simulink model "draft3"  (R2023a)
settings: Solver=VariableStepAuto  StartTime=0.0  StopTime=inf  FixedStep=0.0001  MaxStep=0.2  RelTol=1e-3  AbsTol=1e-3  EnableMultiTasking=on
model workspace (MAT data in the model file):
  c = 0.1
  k : Simulink.Parameter (value not decoded)
libraries: sm_lib x40, nesl_utility x35, simulink_extras x2, fl_lib x1
(part 2 of 3)

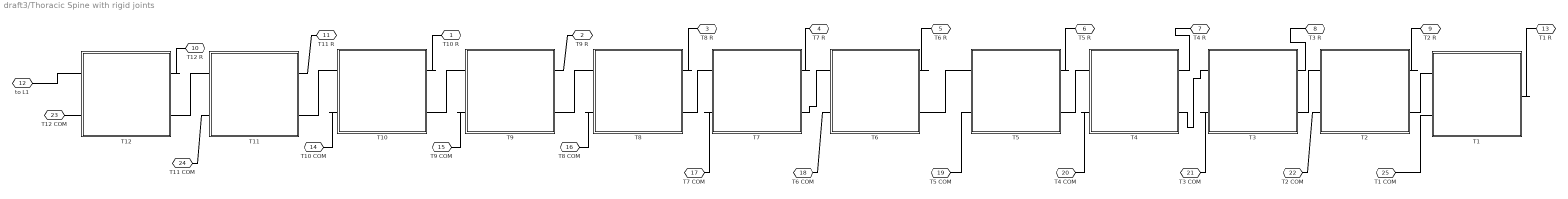
== system draft3/Thoracic Spine with rigid joints ==
  T1 : Subsystem
  T10 : Subsystem
  T11 : Subsystem
  T12 : Subsystem
  T2 : Subsystem
  T3 : Subsystem
  T4 : Subsystem
  T5 : Subsystem
  T6 : Subsystem
  T7 : Subsystem
  T8 : Subsystem
  T9 : Subsystem
  T10 R : PMIOPort  Side=Right
  T9 R : PMIOPort  Port=2  Side=Right
  T8 R : PMIOPort  Port=3  Side=Right
  T7 R : PMIOPort  Port=4  Side=Right
  T6 R : PMIOPort  Port=5  Side=Right
  T5 R : PMIOPort  Port=6  Side=Right
  T4 R : PMIOPort  Port=7  Side=Right
  T3 R : PMIOPort  Port=8  Side=Right
  T2 R : PMIOPort  Port=9  Side=Right
  T12 R : PMIOPort  Port=10  Side=Right
  T11 R : PMIOPort  Port=11  Side=Right
  to L1 : PMIOPort  Port=12  Side=Left
  T1 R : PMIOPort  Port=13  Side=Right
  T10 COM : PMIOPort  Port=14  Side=Left
  T9 COM : PMIOPort  Port=15  Side=Left
  T8 COM : PMIOPort  Port=16  Side=Left
  T7 COM : PMIOPort  Port=17  Side=Left
  T6 COM : PMIOPort  Port=18  Side=Left
  T5 COM : PMIOPort  Port=19  Side=Left
  T4 COM : PMIOPort  Port=20  Side=Left
  T3 COM : PMIOPort  Port=21  Side=Left
  T2 COM : PMIOPort  Port=22  Side=Left
  T12 COM : PMIOPort  Port=23  Side=Left
  T11 COM : PMIOPort  Port=24  Side=Left
  T1 COM : PMIOPort  Port=25  Side=Left
  connections:
  T4/LConn2 -- T4 COM/RConn1
  T7/LConn1 -- T8/RConn2
  T7/LConn2 -- T7 COM/RConn1
  T11/LConn2 -- T11 COM/RConn1
  T1/LConn1 -- T2/RConn2
  T8/LConn1 -- T9/RConn2
  T9/RConn1 -- T9 R/RConn1
  T11/RConn1 -- T11 R/RConn1
  T10/LConn1 -- T11/RConn2
  T5/LConn1 -- T6/RConn2
  T9/LConn1 -- T10/RConn2
  T12/RConn1 -- T12 R/RConn1
  T11/LConn1 -- T12/RConn2
  T1/LConn2 -- T1 COM/RConn1
  T8/LConn2 -- T8 COM/RConn1
  T5/LConn2 -- T5 COM/RConn1
  T6/LConn1 -- T7/RConn2
  T2/LConn2 -- T2 COM/RConn1
  T4/RConn2 -- T3/LConn1
  T10/RConn1 -- T10 R/RConn1
  T2/LConn1 -- T3/RConn2
  T1/RConn1 -- T1 R/RConn1
  T4/LConn1 -- T5/RConn2
  T3/LConn2 -- T3 COM/RConn1
  T12/LConn1 -- to L1/RConn1
  T3/RConn1 -- T3 R/RConn1
  T5/RConn1 -- T5 R/RConn1
  T7/RConn1 -- T7 R/RConn1
  T12/LConn2 -- T12 COM/RConn1
  T2/RConn1 -- T2 R/RConn1
  T6/LConn2 -- T6 COM/RConn1
  T6/RConn1 -- T6 R/RConn1
  T10/LConn2 -- T10 COM/RConn1
  T9/LConn2 -- T9 COM/RConn1
  T4/RConn1 -- T4 R/RConn1
  T8/RConn1 -- T8 R/RConn1

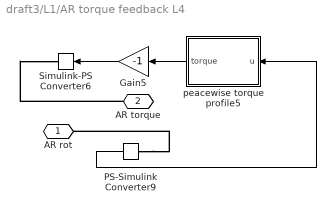
== system draft3/L1/AR torque feedback L4 ==
  Gain5 : Gain  Gain=-1
  PS-Simulink Converter9 : nesl_utility/PS-Simulink Converter  PhysicalDomain=network_engine_domain  SubClassName=ps_output  LeftPortType=input  RightPortType=output  PseudoPeriodic=off  Frequencies=[]  VectorFormat=1-D array  Unit=inherit  AffineConversion=off
  Simulink-PS Converter6 : nesl_utility/Simulink-PS Converter  PhysicalDomain=network_engine_domain  SubClassName=ps_input  LeftPortType=input  RightPortType=output  PseudoPeriodic=off  Frequencies=[]  NoiseDistribution=none  NoiseParameters=[]  Unit=1  AffineConversion=off  FilteringAndDerivatives=provide  SimscapeFilterOrder=1  InputFilterTimeConstant=0.001  UdotUserProvided=0
  peacewise torque profile5 : MATLAB Function  TreatAsAtomicUnit=on
  AR rot : PMIOPort  Side=Left
  AR torque : PMIOPort  Port=2  Side=Right
  wires:
  PS-Simulink Converter9/1 -> peacewise torque profile5/1(u)
  peacewise torque profile5/1(torque) -> Gain5/1
  Gain5/1 -> Simulink-PS Converter6/1
  connections:
  PS-Simulink Converter9/LConn1 -- AR rot/RConn1
  AR torque/RConn1 -- Simulink-PS Converter6/RConn1

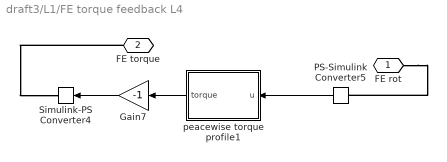
== system draft3/L1/FE torque feedback L4 ==
  Gain7 : Gain  Gain=-1
  PS-Simulink Converter5 : nesl_utility/PS-Simulink Converter  PhysicalDomain=network_engine_domain  SubClassName=ps_output  LeftPortType=input  RightPortType=output  PseudoPeriodic=off  Frequencies=[]  VectorFormat=1-D array  Unit=inherit  AffineConversion=off
  Simulink-PS Converter4 : nesl_utility/Simulink-PS Converter  PhysicalDomain=network_engine_domain  SubClassName=ps_input  LeftPortType=input  RightPortType=output  PseudoPeriodic=off  Frequencies=[]  NoiseDistribution=none  NoiseParameters=[]  Unit=1  AffineConversion=off  FilteringAndDerivatives=provide  SimscapeFilterOrder=1  InputFilterTimeConstant=0.001  UdotUserProvided=0
  peacewise torque profile1 : MATLAB Function  TreatAsAtomicUnit=on
  FE rot : PMIOPort  Side=Left
  FE torque : PMIOPort  Port=2  Side=Right
  wires:
  PS-Simulink Converter5/1 -> peacewise torque profile1/1(u)
  peacewise torque profile1/1(torque) -> Gain7/1
  Gain7/1 -> Simulink-PS Converter4/1
  connections:
  FE rot/RConn1 -- PS-Simulink Converter5/LConn1
  FE torque/RConn1 -- Simulink-PS Converter4/RConn1

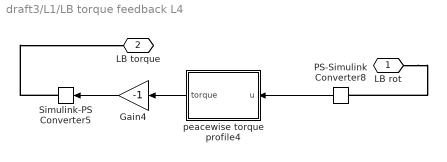
== system draft3/L1/LB torque feedback L4 ==
  Gain4 : Gain  Gain=-1
  PS-Simulink Converter8 : nesl_utility/PS-Simulink Converter  PhysicalDomain=network_engine_domain  SubClassName=ps_output  LeftPortType=input  RightPortType=output  PseudoPeriodic=off  Frequencies=[]  VectorFormat=1-D array  Unit=inherit  AffineConversion=off
  Simulink-PS Converter5 : nesl_utility/Simulink-PS Converter  PhysicalDomain=network_engine_domain  SubClassName=ps_input  LeftPortType=input  RightPortType=output  PseudoPeriodic=off  Frequencies=[]  NoiseDistribution=none  NoiseParameters=[]  Unit=1  AffineConversion=off  FilteringAndDerivatives=provide  SimscapeFilterOrder=1  InputFilterTimeConstant=0.001  UdotUserProvided=0
  peacewise torque profile4 : MATLAB Function  TreatAsAtomicUnit=on
  LB rot : PMIOPort  Side=Left
  LB torque : PMIOPort  Port=2  Side=Right
  wires:
  Gain4/1 -> Simulink-PS Converter5/1
  PS-Simulink Converter8/1 -> peacewise torque profile4/1(u)
  peacewise torque profile4/1(torque) -> Gain4/1
  connections:
  Simulink-PS Converter5/RConn1 -- LB torque/RConn1
  LB rot/RConn1 -- PS-Simulink Converter8/LConn1

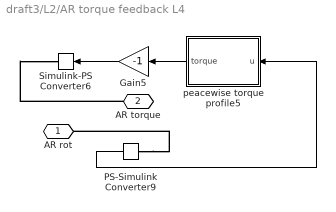
== system draft3/L2/AR torque feedback L4 ==
  Gain5 : Gain  Gain=-1
  PS-Simulink Converter9 : nesl_utility/PS-Simulink Converter  PhysicalDomain=network_engine_domain  SubClassName=ps_output  LeftPortType=input  RightPortType=output  PseudoPeriodic=off  Frequencies=[]  VectorFormat=1-D array  Unit=inherit  AffineConversion=off
  Simulink-PS Converter6 : nesl_utility/Simulink-PS Converter  PhysicalDomain=network_engine_domain  SubClassName=ps_input  LeftPortType=input  RightPortType=output  PseudoPeriodic=off  Frequencies=[]  NoiseDistribution=none  NoiseParameters=[]  Unit=1  AffineConversion=off  FilteringAndDerivatives=provide  SimscapeFilterOrder=1  InputFilterTimeConstant=0.001  UdotUserProvided=0
  peacewise torque profile5 : MATLAB Function  TreatAsAtomicUnit=on
  AR rot : PMIOPort  Side=Left
  AR torque : PMIOPort  Port=2  Side=Right
  wires:
  Gain5/1 -> Simulink-PS Converter6/1
  peacewise torque profile5/1(torque) -> Gain5/1
  PS-Simulink Converter9/1 -> peacewise torque profile5/1(u)
  connections:
  AR torque/RConn1 -- Simulink-PS Converter6/RConn1
  PS-Simulink Converter9/LConn1 -- AR rot/RConn1

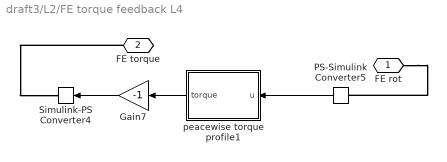
== system draft3/L2/FE torque feedback L4 ==
  Gain7 : Gain  Gain=-1
  PS-Simulink Converter5 : nesl_utility/PS-Simulink Converter  PhysicalDomain=network_engine_domain  SubClassName=ps_output  LeftPortType=input  RightPortType=output  PseudoPeriodic=off  Frequencies=[]  VectorFormat=1-D array  Unit=inherit  AffineConversion=off
  Simulink-PS Converter4 : nesl_utility/Simulink-PS Converter  PhysicalDomain=network_engine_domain  SubClassName=ps_input  LeftPortType=input  RightPortType=output  PseudoPeriodic=off  Frequencies=[]  NoiseDistribution=none  NoiseParameters=[]  Unit=1  AffineConversion=off  FilteringAndDerivatives=provide  SimscapeFilterOrder=1  InputFilterTimeConstant=0.001  UdotUserProvided=0
  peacewise torque profile1 : MATLAB Function  TreatAsAtomicUnit=on
  FE rot : PMIOPort  Side=Left
  FE torque : PMIOPort  Port=2  Side=Right
  wires:
  Gain7/1 -> Simulink-PS Converter4/1
  peacewise torque profile1/1(torque) -> Gain7/1
  PS-Simulink Converter5/1 -> peacewise torque profile1/1(u)
  connections:
  FE torque/RConn1 -- Simulink-PS Converter4/RConn1
  FE rot/RConn1 -- PS-Simulink Converter5/LConn1

== system draft3/L2/LB torque feedback L4 ==
  Gain4 : Gain  Gain=-1
  PS-Simulink Converter8 : nesl_utility/PS-Simulink Converter  PhysicalDomain=network_engine_domain  SubClassName=ps_output  LeftPortType=input  RightPortType=output  PseudoPeriodic=off  Frequencies=[]  VectorFormat=1-D array  Unit=inherit  AffineConversion=off
  Simulink-PS Converter5 : nesl_utility/Simulink-PS Converter  PhysicalDomain=network_engine_domain  SubClassName=ps_input  LeftPortType=input  RightPortType=output  PseudoPeriodic=off  Frequencies=[]  NoiseDistribution=none  NoiseParameters=[]  Unit=1  AffineConversion=off  FilteringAndDerivatives=provide  SimscapeFilterOrder=1  InputFilterTimeConstant=0.001  UdotUserProvided=0
  peacewise torque profile4 : MATLAB Function  TreatAsAtomicUnit=on
  LB rot : PMIOPort  Side=Left
  LB torque : PMIOPort  Port=2  Side=Right
  wires:
  peacewise torque profile4/1(torque) -> Gain4/1
  PS-Simulink Converter8/1 -> peacewise torque profile4/1(u)
  Gain4/1 -> Simulink-PS Converter5/1
  connections:
  LB rot/RConn1 -- PS-Simulink Converter8/LConn1
  Simulink-PS Converter5/RConn1 -- LB torque/RConn1

== system draft3/L3/AR torque feedback L4 ==
  Gain5 : Gain  Gain=-1
  PS-Simulink Converter9 : nesl_utility/PS-Simulink Converter  PhysicalDomain=network_engine_domain  SubClassName=ps_output  LeftPortType=input  RightPortType=output  PseudoPeriodic=off  Frequencies=[]  VectorFormat=1-D array  Unit=inherit  AffineConversion=off
  Simulink-PS Converter6 : nesl_utility/Simulink-PS Converter  PhysicalDomain=network_engine_domain  SubClassName=ps_input  LeftPortType=input  RightPortType=output  PseudoPeriodic=off  Frequencies=[]  NoiseDistribution=none  NoiseParameters=[]  Unit=1  AffineConversion=off  FilteringAndDerivatives=provide  SimscapeFilterOrder=1  InputFilterTimeConstant=0.001  UdotUserProvided=0
  peacewise torque profile5 : MATLAB Function  TreatAsAtomicUnit=on
  AR rot : PMIOPort  Side=Left
  AR torque : PMIOPort  Port=2  Side=Right
  wires:
  PS-Simulink Converter9/1 -> peacewise torque profile5/1(u)
  peacewise torque profile5/1(torque) -> Gain5/1
  Gain5/1 -> Simulink-PS Converter6/1
  connections:
  PS-Simulink Converter9/LConn1 -- AR rot/RConn1
  AR torque/RConn1 -- Simulink-PS Converter6/RConn1

== system draft3/L3/FE torque feedback L4 ==
  Gain7 : Gain  Gain=-1
  PS-Simulink Converter5 : nesl_utility/PS-Simulink Converter  PhysicalDomain=network_engine_domain  SubClassName=ps_output  LeftPortType=input  RightPortType=output  PseudoPeriodic=off  Frequencies=[]  VectorFormat=1-D array  Unit=inherit  AffineConversion=off
  Simulink-PS Converter4 : nesl_utility/Simulink-PS Converter  PhysicalDomain=network_engine_domain  SubClassName=ps_input  LeftPortType=input  RightPortType=output  PseudoPeriodic=off  Frequencies=[]  NoiseDistribution=none  NoiseParameters=[]  Unit=1  AffineConversion=off  FilteringAndDerivatives=provide  SimscapeFilterOrder=1  InputFilterTimeConstant=0.001  UdotUserProvided=0
  peacewise torque profile1 : MATLAB Function  TreatAsAtomicUnit=on
  FE rot : PMIOPort  Side=Left
  FE torque : PMIOPort  Port=2  Side=Right
  wires:
  PS-Simulink Converter5/1 -> peacewise torque profile1/1(u)
  peacewise torque profile1/1(torque) -> Gain7/1
  Gain7/1 -> Simulink-PS Converter4/1
  connections:
  FE rot/RConn1 -- PS-Simulink Converter5/LConn1
  FE torque/RConn1 -- Simulink-PS Converter4/RConn1

== system draft3/L3/LB torque feedback L4 ==
  Gain4 : Gain  Gain=-1
  PS-Simulink Converter8 : nesl_utility/PS-Simulink Converter  PhysicalDomain=network_engine_domain  SubClassName=ps_output  LeftPortType=input  RightPortType=output  PseudoPeriodic=off  Frequencies=[]  VectorFormat=1-D array  Unit=inherit  AffineConversion=off
  Simulink-PS Converter5 : nesl_utility/Simulink-PS Converter  PhysicalDomain=network_engine_domain  SubClassName=ps_input  LeftPortType=input  RightPortType=output  PseudoPeriodic=off  Frequencies=[]  NoiseDistribution=none  NoiseParameters=[]  Unit=1  AffineConversion=off  FilteringAndDerivatives=provide  SimscapeFilterOrder=1  InputFilterTimeConstant=0.001  UdotUserProvided=0
  peacewise torque profile4 : MATLAB Function  TreatAsAtomicUnit=on
  LB rot : PMIOPort  Side=Left
  LB torque : PMIOPort  Port=2  Side=Right
  wires:
  Gain4/1 -> Simulink-PS Converter5/1
  PS-Simulink Converter8/1 -> peacewise torque profile4/1(u)
  peacewise torque profile4/1(torque) -> Gain4/1
  connections:
  Simulink-PS Converter5/RConn1 -- LB torque/RConn1
  LB rot/RConn1 -- PS-Simulink Converter8/LConn1

== system draft3/L4/AR torque feedback L4 ==
  Gain5 : Gain  Gain=-1
  PS-Simulink Converter9 : nesl_utility/PS-Simulink Converter  PhysicalDomain=network_engine_domain  SubClassName=ps_output  LeftPortType=input  RightPortType=output  PseudoPeriodic=off  Frequencies=[]  VectorFormat=1-D array  Unit=inherit  AffineConversion=off
  Simulink-PS Converter6 : nesl_utility/Simulink-PS Converter  PhysicalDomain=network_engine_domain  SubClassName=ps_input  LeftPortType=input  RightPortType=output  PseudoPeriodic=off  Frequencies=[]  NoiseDistribution=none  NoiseParameters=[]  Unit=1  AffineConversion=off  FilteringAndDerivatives=provide  SimscapeFilterOrder=1  InputFilterTimeConstant=0.001  UdotUserProvided=0
  peacewise torque profile5 : MATLAB Function  TreatAsAtomicUnit=on
  AR rot : PMIOPort  Side=Left
  AR torque : PMIOPort  Port=2  Side=Right
  wires:
  Gain5/1 -> Simulink-PS Converter6/1
  peacewise torque profile5/1(torque) -> Gain5/1
  PS-Simulink Converter9/1 -> peacewise torque profile5/1(u)
  connections:
  AR torque/RConn1 -- Simulink-PS Converter6/RConn1
  PS-Simulink Converter9/LConn1 -- AR rot/RConn1

== system draft3/L4/FE torque feedback L4 ==
  Gain7 : Gain  Gain=-1
  PS-Simulink Converter5 : nesl_utility/PS-Simulink Converter  PhysicalDomain=network_engine_domain  SubClassName=ps_output  LeftPortType=input  RightPortType=output  PseudoPeriodic=off  Frequencies=[]  VectorFormat=1-D array  Unit=inherit  AffineConversion=off
  Simulink-PS Converter4 : nesl_utility/Simulink-PS Converter  PhysicalDomain=network_engine_domain  SubClassName=ps_input  LeftPortType=input  RightPortType=output  PseudoPeriodic=off  Frequencies=[]  NoiseDistribution=none  NoiseParameters=[]  Unit=1  AffineConversion=off  FilteringAndDerivatives=provide  SimscapeFilterOrder=1  InputFilterTimeConstant=0.001  UdotUserProvided=0
  peacewise torque profile1 : MATLAB Function  TreatAsAtomicUnit=on
  FE rot : PMIOPort  Side=Left
  FE torque : PMIOPort  Port=2  Side=Right
  wires:
  Gain7/1 -> Simulink-PS Converter4/1
  peacewise torque profile1/1(torque) -> Gain7/1
  PS-Simulink Converter5/1 -> peacewise torque profile1/1(u)
  connections:
  FE torque/RConn1 -- Simulink-PS Converter4/RConn1
  FE rot/RConn1 -- PS-Simulink Converter5/LConn1

== system draft3/L4/LB torque feedback L4 ==
  Gain4 : Gain  Gain=-1
  PS-Simulink Converter8 : nesl_utility/PS-Simulink Converter  PhysicalDomain=network_engine_domain  SubClassName=ps_output  LeftPortType=input  RightPortType=output  PseudoPeriodic=off  Frequencies=[]  VectorFormat=1-D array  Unit=inherit  AffineConversion=off
  Simulink-PS Converter5 : nesl_utility/Simulink-PS Converter  PhysicalDomain=network_engine_domain  SubClassName=ps_input  LeftPortType=input  RightPortType=output  PseudoPeriodic=off  Frequencies=[]  NoiseDistribution=none  NoiseParameters=[]  Unit=1  AffineConversion=off  FilteringAndDerivatives=provide  SimscapeFilterOrder=1  InputFilterTimeConstant=0.001  UdotUserProvided=0
  peacewise torque profile4 : MATLAB Function  TreatAsAtomicUnit=on
  LB rot : PMIOPort  Side=Left
  LB torque : PMIOPort  Port=2  Side=Right
  wires:
  peacewise torque profile4/1(torque) -> Gain4/1
  PS-Simulink Converter8/1 -> peacewise torque profile4/1(u)
  Gain4/1 -> Simulink-PS Converter5/1
  connections:
  LB rot/RConn1 -- PS-Simulink Converter8/LConn1
  Simulink-PS Converter5/RConn1 -- LB torque/RConn1

== system draft3/L5/AR torque feedback L5 ==
  Gain2 : Gain  Gain=-1
  PS-Simulink Converter3 : nesl_utility/PS-Simulink Converter  PhysicalDomain=network_engine_domain  SubClassName=ps_output  LeftPortType=input  RightPortType=output  PseudoPeriodic=off  Frequencies=[]  VectorFormat=1-D array  Unit=inherit  AffineConversion=off
  Simulink-PS Converter2 : nesl_utility/Simulink-PS Converter  PhysicalDomain=network_engine_domain  SubClassName=ps_input  LeftPortType=input  RightPortType=output  PseudoPeriodic=off  Frequencies=[]  NoiseDistribution=none  NoiseParameters=[]  Unit=1  AffineConversion=off  FilteringAndDerivatives=provide  SimscapeFilterOrder=1  InputFilterTimeConstant=0.001  UdotUserProvided=0
  peacewise torque profile3 : MATLAB Function  TreatAsAtomicUnit=on
  AR rot : PMIOPort  Side=Left
  AR torque : PMIOPort  Port=2  Side=Right
  wires:
  peacewise torque profile3/1(torque) -> Gain2/1
  Gain2/1 -> Simulink-PS Converter2/1
  PS-Simulink Converter3/1 -> peacewise torque profile3/1(u)
  connections:
  AR torque/RConn1 -- Simulink-PS Converter2/RConn1
  PS-Simulink Converter3/LConn1 -- AR rot/RConn1

== system draft3/L5/FE torque feedback L5 ==
  Gain6 : Gain  Gain=-1
  PS-Simulink Converter1 : nesl_utility/PS-Simulink Converter  PhysicalDomain=network_engine_domain  SubClassName=ps_output  LeftPortType=input  RightPortType=output  PseudoPeriodic=off  Frequencies=[]  VectorFormat=1-D array  Unit=inherit  AffineConversion=off
  Simulink-PS Converter3 : nesl_utility/Simulink-PS Converter  PhysicalDomain=network_engine_domain  SubClassName=ps_input  LeftPortType=input  RightPortType=output  PseudoPeriodic=off  Frequencies=[]  NoiseDistribution=none  NoiseParameters=[]  Unit=1  AffineConversion=off  FilteringAndDerivatives=provide  SimscapeFilterOrder=1  InputFilterTimeConstant=0.001  UdotUserProvided=0
  peacewise torque profile (+- 15 deg) : MATLAB Function  TreatAsAtomicUnit=on
  FE torque : PMIOPort  Side=Right
  FE rot : PMIOPort  Port=2  Side=Left
  wires:
  Gain6/1 -> Simulink-PS Converter3/1
  PS-Simulink Converter1/1 -> peacewise torque profile (+- 15 deg)/1(u)
  peacewise torque profile (+- 15 deg)/1(torque) -> Gain6/1
  connections:
  PS-Simulink Converter1/LConn1 -- FE rot/RConn1
  Simulink-PS Converter3/RConn1 -- FE torque/RConn1

== system draft3/L5/LB torque feedback L5 ==
  Gain1 : Gain  Gain=-1
  PS-Simulink Converter2 : nesl_utility/PS-Simulink Converter  PhysicalDomain=network_engine_domain  SubClassName=ps_output  LeftPortType=input  RightPortType=output  PseudoPeriodic=off  Frequencies=[]  VectorFormat=1-D array  Unit=inherit  AffineConversion=off
  Simulink-PS Converter1 : nesl_utility/Simulink-PS Converter  PhysicalDomain=network_engine_domain  SubClassName=ps_input  LeftPortType=input  RightPortType=output  PseudoPeriodic=off  Frequencies=[]  NoiseDistribution=none  NoiseParameters=[]  Unit=1  AffineConversion=off  FilteringAndDerivatives=provide  SimscapeFilterOrder=1  InputFilterTimeConstant=0.001  UdotUserProvided=0
  peacewise torque profile2 : MATLAB Function  TreatAsAtomicUnit=on
  LB rot : PMIOPort  Side=Left
  LB torque : PMIOPort  Port=2  Side=Right
  wires:
  Gain1/1 -> Simulink-PS Converter1/1
  PS-Simulink Converter2/1 -> peacewise torque profile2/1(u)
  peacewise torque profile2/1(torque) -> Gain1/1
  connections:
  LB rot/RConn1 -- PS-Simulink Converter2/LConn1
  Simulink-PS Converter1/RConn1 -- LB torque/RConn1

== system draft3/Thoracic Spine with rigid joints/T1 ==
  T1 : sm_lib/Body Elements/File Solid  ExtGeomFileName=C:\Users\siril\OneDrive\Desktop\TIM-Control\Matlab\Simscape models\CAD - with COM\T1_.step  UnitType=FromFile  ExtGeomFileUnits=m  StepReaderType=HEX  ExportConvexHullGeometry=off  InertiaType=CalculateFromGeometry  Mass=1  MassUnits=kg  CenterOfMass=[0 0 0]  CenterOfMassUnits=m  MomentsOfInertia=[1 1 1]  MomentsOfInertiaUnits=kg*m^2  ProductsOfInertia=[0 0 0]  ProductsOfInertiaUnits=kg*m^2  BasedOnType=Density  Density=0.99  DensityUnits=g/cm^3  DoExposeReferenceFrame=on  SerializedFrames=<Frames><Frame><Id>Frame1</Id><Value><Name>COM</Name><Origin><Source>CenterOfMassFrame</Source><FeatureName></FeatureName></Origin><PrimaryAxis><DefinedDirection>+Z</DefinedDirection><Source>ReferenceFrame</Source><SourceDirection>+Z</SourceDirection><FeatureName></FeatureName></PrimaryAxis><SecondaryAxis><DefinedDirection>+X</DefinedDirection><Source>ReferenceFrame</Source><SourceDirection>+X</SourceDirection><FeatureName></FeatureName></SecondaryAxis></Value></Frame><Frame><Id>Frame2</Id><Value><Name>to T2</Name><Origin><Source>GeometricFeature</Source><FeatureName>planar surface 5</FeatureName></Origin><PrimaryAxis><DefinedDirection>+X</DefinedDirection><Source>GeometricFeature</Source><SourceDirection>+Z</SourceDirection><FeatureName>planar surface 5</FeatureName></PrimaryAxis><SecondaryAxis><DefinedDirection>+Y</DefinedDirection><Source>ReferenceFrame</Source><SourceDirection>+X</SourceDirection><FeatureName></FeatureName></SecondaryAxis></Value></Frame></Frames>  GraphicType=FromGeometry  MarkerShape=Sphere  MarkerSize=10  GraphicVisPropType=SimpleVisualProperties  GraphicDiffuseColor=[0.5 0.5 0.5]  GraphicSpecularColor=[0.5 0.5 0.5 1.0]  GraphicAmbientColor=[0.15 0.15 0.15 1.0]  GraphicEmissiveColor=[0.0 0.0 0.0 1.0]  GraphicShininess=75  GraphicOpacity=1.0
  Weld Joint : sm_lib/Joints/Weld Joint  JointMode=Normal  SenseConstraintForce=off  SenseConstraintForceX=off  SenseConstraintForceY=off  SenseConstraintForceZ=off  SenseConstraintTorque=off  SenseConstraintTorqueX=off  SenseConstraintTorqueY=off  SenseConstraintTorqueZ=off  SenseTotalForce=off  SenseTotalForceX=off  SenseTotalForceY=off  SenseTotalForceZ=off  SenseTotalTorque=off  SenseTotalTorqueX=off  SenseTotalTorqueY=off  SenseTotalTorqueZ=off  CompositeWrenchDir=FollowerOnBase  CompositeWrenchFrame=BaseFrame
  to T2 : PMIOPort  Side=Left
  T1 COM : PMIOPort  Port=2  Side=Left
  T1 R : PMIOPort  Port=3  Side=Right
  connections:
  Weld Joint/LConn1 -- to T2/RConn1
  T1 COM/RConn1 -- T1/LConn1
  Weld Joint/RConn1 -- T1/LConn2
  T1/RConn1 -- T1 R/RConn1

== system draft3/Thoracic Spine with rigid joints/T10 ==
  T10 : sm_lib/Body Elements/File Solid  ExtGeomFileName=C:\Users\siril\OneDrive\Desktop\TIM-Control\Matlab\Simscape models\CAD - with COM\T10_.step  UnitType=FromFile  ExtGeomFileUnits=m  StepReaderType=HEX  ExportConvexHullGeometry=off  InertiaType=CalculateFromGeometry  Mass=1  MassUnits=kg  CenterOfMass=[0 0 0]  CenterOfMassUnits=m  MomentsOfInertia=[1 1 1]  MomentsOfInertiaUnits=kg*m^2  ProductsOfInertia=[0 0 0]  ProductsOfInertiaUnits=kg*m^2  BasedOnType=Density  Density=0.99  DensityUnits=g/cm^3  DoExposeReferenceFrame=on  SerializedFrames=<Frames><Frame><Id>Frame1</Id><Value><Name>COM</Name><Origin><Source>CenterOfMassFrame</Source><FeatureName></FeatureName></Origin><PrimaryAxis><DefinedDirection>+Z</DefinedDirection><Source>ReferenceFrame</Source><SourceDirection>+Z</SourceDirection><FeatureName></FeatureName></PrimaryAxis><SecondaryAxis><DefinedDirection>+X</DefinedDirection><Source>ReferenceFrame</Source><SourceDirection>+X</SourceDirection><FeatureName></FeatureName></SecondaryAxis></Value></Frame><Frame><Id>Frame2</Id><Value><Name>to T11</Name><Origin><Source>GeometricFeature</Source><FeatureName>planar surface 5</FeatureName></Origin><PrimaryAxis><DefinedDirection>+X</DefinedDirection><Source>GeometricFeature</Source><SourceDirection>+Z</SourceDirection><FeatureName>planar surface 5</FeatureName></PrimaryAxis><SecondaryAxis><DefinedDirection>+Y</DefinedDirection><Source>ReferenceFrame</Source><SourceDirection>-X</SourceDirection><FeatureName></FeatureName></SecondaryAxis></Value></Frame><Frame><Id>Frame3</Id><Value><Name>to T9</Name><Origin><Source>GeometricFeature</Source><FeatureName>planar surface 12</FeatureName></Origin><PrimaryAxis><DefinedDirection>+X</DefinedDirection><Source>GeometricFeature</Source><SourceDirection>+Z</SourceDirection><FeatureName>planar surface 12</FeatureName></PrimaryAxis><SecondaryAxis><DefinedDirection>+Y</DefinedDirection><Source>ReferenceFrame</Source><SourceDirection>-X</SourceDirection><FeatureName></FeatureName></SecondaryAxis></Value></Frame></Frames>  GraphicType=FromGeometry  MarkerShape=Sphere  MarkerSize=10  GraphicVisPropType=SimpleVisualProperties  GraphicDiffuseColor=[0.5 0.5 0.5]  GraphicSpecularColor=[0.5 0.5 0.5 1.0]  GraphicAmbientColor=[0.15 0.15 0.15 1.0]  GraphicEmissiveColor=[0.0 0.0 0.0 1.0]  GraphicShininess=75  GraphicOpacity=1.0
  Weld Joint : sm_lib/Joints/Weld Joint  JointMode=Normal  SenseConstraintForce=off  SenseConstraintForceX=off  SenseConstraintForceY=off  SenseConstraintForceZ=off  SenseConstraintTorque=off  SenseConstraintTorqueX=off  SenseConstraintTorqueY=off  SenseConstraintTorqueZ=off  SenseTotalForce=off  SenseTotalForceX=off  SenseTotalForceY=off  SenseTotalForceZ=off  SenseTotalTorque=off  SenseTotalTorqueX=off  SenseTotalTorqueY=off  SenseTotalTorqueZ=off  CompositeWrenchDir=FollowerOnBase  CompositeWrenchFrame=BaseFrame
  to T11 : PMIOPort  Side=Left
  T10 COM : PMIOPort  Port=2  Side=Left
  T10 R : PMIOPort  Port=3  Side=Right
  to T9 : PMIOPort  Port=4  Side=Right
  connections:
  to T9/RConn1 -- T10/RConn2
  T10/RConn1 -- T10 R/RConn1
  T10 COM/RConn1 -- T10/LConn1
  to T11/RConn1 -- Weld Joint/LConn1
  Weld Joint/RConn1 -- T10/LConn2

== system draft3/Thoracic Spine with rigid joints/T11 ==
  T11 : sm_lib/Body Elements/File Solid  ExtGeomFileName=C:\Users\siril\OneDrive\Desktop\TIM-Control\Matlab\Simscape models\CAD - with COM\T11_.step  UnitType=FromFile  ExtGeomFileUnits=m  StepReaderType=HEX  ExportConvexHullGeometry=off  InertiaType=CalculateFromGeometry  Mass=1  MassUnits=kg  CenterOfMass=[0 0 0]  CenterOfMassUnits=m  MomentsOfInertia=[1 1 1]  MomentsOfInertiaUnits=kg*m^2  ProductsOfInertia=[0 0 0]  ProductsOfInertiaUnits=kg*m^2  BasedOnType=Density  Density=0.99  DensityUnits=g/cm^3  DoExposeReferenceFrame=on  SerializedFrames=<Frames><Frame><Id>Frame1</Id><Value><Name>COM</Name><Origin><Source>CenterOfMassFrame</Source><FeatureName></FeatureName></Origin><PrimaryAxis><DefinedDirection>+Z</DefinedDirection><Source>ReferenceFrame</Source><SourceDirection>+Z</SourceDirection><FeatureName></FeatureName></PrimaryAxis><SecondaryAxis><DefinedDirection>+X</DefinedDirection><Source>ReferenceFrame</Source><SourceDirection>+X</SourceDirection><FeatureName></FeatureName></SecondaryAxis></Value></Frame><Frame><Id>Frame2</Id><Value><Name>to T12</Name><Origin><Source>GeometricFeature</Source><FeatureName>planar surface 5</FeatureName></Origin><PrimaryAxis><DefinedDirection>+X</DefinedDirection><Source>GeometricFeature</Source><SourceDirection>+Z</SourceDirection><FeatureName>planar surface 5</FeatureName></PrimaryAxis><SecondaryAxis><DefinedDirection>+Y</DefinedDirection><Source>ReferenceFrame</Source><SourceDirection>-X</SourceDirection><FeatureName></FeatureName></SecondaryAxis></Value></Frame><Frame><Id>Frame3</Id><Value><Name>to T10</Name><Origin><Source>GeometricFeature</Source><FeatureName>planar surface 12</FeatureName></Origin><PrimaryAxis><DefinedDirection>+X</DefinedDirection><Source>GeometricFeature</Source><SourceDirection>+Z</SourceDirection><FeatureName>planar surface 12</FeatureName></PrimaryAxis><SecondaryAxis><DefinedDirection>+Y</DefinedDirection><Source>ReferenceFrame</Source><SourceDirection>-X</SourceDirection><FeatureName></FeatureName></SecondaryAxis></Value></Frame></Frames>  GraphicType=FromGeometry  MarkerShape=Sphere  MarkerSize=10  GraphicVisPropType=SimpleVisualProperties  GraphicDiffuseColor=[0.5 0.5 0.5]  GraphicSpecularColor=[0.5 0.5 0.5 1.0]  GraphicAmbientColor=[0.15 0.15 0.15 1.0]  GraphicEmissiveColor=[0.0 0.0 0.0 1.0]  GraphicShininess=75  GraphicOpacity=1.0
  Weld Joint : sm_lib/Joints/Weld Joint  JointMode=Normal  SenseConstraintForce=off  SenseConstraintForceX=off  SenseConstraintForceY=off  SenseConstraintForceZ=off  SenseConstraintTorque=off  SenseConstraintTorqueX=off  SenseConstraintTorqueY=off  SenseConstraintTorqueZ=off  SenseTotalForce=off  SenseTotalForceX=off  SenseTotalForceY=off  SenseTotalForceZ=off  SenseTotalTorque=off  SenseTotalTorqueX=off  SenseTotalTorqueY=off  SenseTotalTorqueZ=off  CompositeWrenchDir=FollowerOnBase  CompositeWrenchFrame=BaseFrame
  to T12 : PMIOPort  Side=Left
  T11 COM : PMIOPort  Port=2  Side=Left
  T11 R : PMIOPort  Port=3  Side=Right
  to T10 : PMIOPort  Port=4  Side=Right
  connections:
  T11 COM/RConn1 -- T11/LConn1
  T11/RConn1 -- T11 R/RConn1
  to T10/RConn1 -- T11/RConn2
  to T12/RConn1 -- Weld Joint/LConn1
  Weld Joint/RConn1 -- T11/LConn2

== system draft3/Thoracic Spine with rigid joints/T12 ==
  T12 : sm_lib/Body Elements/File Solid  ExtGeomFileName=C:\Users\siril\OneDrive\Desktop\TIM-Control\Matlab\Simscape models\CAD - with COM\T12_.step  UnitType=FromFile  ExtGeomFileUnits=m  StepReaderType=HEX  ExportConvexHullGeometry=off  InertiaType=CalculateFromGeometry  Mass=1  MassUnits=kg  CenterOfMass=[0 0 0]  CenterOfMassUnits=m  MomentsOfInertia=[1 1 1]  MomentsOfInertiaUnits=kg*m^2  ProductsOfInertia=[0 0 0]  ProductsOfInertiaUnits=kg*m^2  BasedOnType=Density  Density=0.99  DensityUnits=g/cm^3  DoExposeReferenceFrame=on  SerializedFrames=<Frames><Frame><Id>Frame1</Id><Value><Name>COM</Name><Origin><Source>CenterOfMassFrame</Source><FeatureName></FeatureName></Origin><PrimaryAxis><DefinedDirection>+Z</DefinedDirection><Source>ReferenceFrame</Source><SourceDirection>+Z</SourceDirection><FeatureName></FeatureName></PrimaryAxis><SecondaryAxis><DefinedDirection>+X</DefinedDirection><Source>ReferenceFrame</Source><SourceDirection>+X</SourceDirection><FeatureName></FeatureName></SecondaryAxis></Value></Frame><Frame><Id>Frame2</Id><Value><Name>to L1</Name><Origin><Source>GeometricFeature</Source><FeatureName>planar surface 6</FeatureName></Origin><PrimaryAxis><DefinedDirection>+X</DefinedDirection><Source>GeometricFeature</Source><SourceDirection>+Z</SourceDirection><FeatureName>planar surface 6</FeatureName></PrimaryAxis><SecondaryAxis><DefinedDirection>+Y</DefinedDirection><Source>ReferenceFrame</Source><SourceDirection>-X</SourceDirection><FeatureName></FeatureName></SecondaryAxis></Value></Frame><Frame><Id>Frame3</Id><Value><Name>to T11</Name><Origin><Source>GeometricFeature</Source><FeatureName>planar surface 13</FeatureName></Origin><PrimaryAxis><DefinedDirection>+X</DefinedDirection><Source>GeometricFeature</Source><SourceDirection>+Z</SourceDirection><FeatureName>planar surface 13</FeatureName></PrimaryAxis><SecondaryAxis><DefinedDirection>+Y</DefinedDirection><Source>ReferenceFrame</Source><SourceDirection>-X</SourceDirection><FeatureName></FeatureName></SecondaryAxis></Value></Frame></Frames>  GraphicType=FromGeometry  MarkerShape=Sphere  MarkerSize=10  GraphicVisPropType=SimpleVisualProperties  GraphicDiffuseColor=[0.5 0.5 0.5]  GraphicSpecularColor=[0.5 0.5 0.5 1.0]  GraphicAmbientColor=[0.15 0.15 0.15 1.0]  GraphicEmissiveColor=[0.0 0.0 0.0 1.0]  GraphicShininess=75  GraphicOpacity=1.0
  Weld Joint : sm_lib/Joints/Weld Joint  JointMode=Normal  SenseConstraintForce=off  SenseConstraintForceX=off  SenseConstraintForceY=off  SenseConstraintForceZ=off  SenseConstraintTorque=off  SenseConstraintTorqueX=off  SenseConstraintTorqueY=off  SenseConstraintTorqueZ=off  SenseTotalForce=off  SenseTotalForceX=off  SenseTotalForceY=off  SenseTotalForceZ=off  SenseTotalTorque=off  SenseTotalTorqueX=off  SenseTotalTorqueY=off  SenseTotalTorqueZ=off  CompositeWrenchDir=FollowerOnBase  CompositeWrenchFrame=BaseFrame
  to L1 : PMIOPort  Side=Left
  T12 COM : PMIOPort  Port=2  Side=Left
  T12 R : PMIOPort  Port=3  Side=Right
  to T11 : PMIOPort  Port=4  Side=Right
  connections:
  to T11/RConn1 -- T12/RConn2
  T12/RConn1 -- T12 R/RConn1
  T12 COM/RConn1 -- T12/LConn1
  to L1/RConn1 -- Weld Joint/LConn1
  Weld Joint/RConn1 -- T12/LConn2

== system draft3/Thoracic Spine with rigid joints/T2 ==
  T2 : sm_lib/Body Elements/File Solid  ExtGeomFileName=C:\Users\siril\OneDrive\Desktop\TIM-Control\Matlab\Simscape models\CAD - with COM\T2_.step  UnitType=FromFile  ExtGeomFileUnits=m  StepReaderType=HEX  ExportConvexHullGeometry=off  InertiaType=CalculateFromGeometry  Mass=1  MassUnits=kg  CenterOfMass=[0 0 0]  CenterOfMassUnits=m  MomentsOfInertia=[1 1 1]  MomentsOfInertiaUnits=kg*m^2  ProductsOfInertia=[0 0 0]  ProductsOfInertiaUnits=kg*m^2  BasedOnType=Density  Density=0.99  DensityUnits=g/cm^3  DoExposeReferenceFrame=on  SerializedFrames=<Frames><Frame><Id>Frame1</Id><Value><Name>COM</Name><Origin><Source>CenterOfMassFrame</Source><FeatureName></FeatureName></Origin><PrimaryAxis><DefinedDirection>+Z</DefinedDirection><Source>ReferenceFrame</Source><SourceDirection>+Z</SourceDirection><FeatureName></FeatureName></PrimaryAxis><SecondaryAxis><DefinedDirection>+X</DefinedDirection><Source>ReferenceFrame</Source><SourceDirection>+X</SourceDirection><FeatureName></FeatureName></SecondaryAxis></Value></Frame><Frame><Id>Frame2</Id><Value><Name>to T3</Name><Origin><Source>GeometricFeature</Source><FeatureName>planar surface 5</FeatureName></Origin><PrimaryAxis><DefinedDirection>+X</DefinedDirection><Source>GeometricFeature</Source><SourceDirection>+Z</SourceDirection><FeatureName>planar surface 5</FeatureName></PrimaryAxis><SecondaryAxis><DefinedDirection>+Y</DefinedDirection><Source>ReferenceFrame</Source><SourceDirection>+X</SourceDirection><FeatureName></FeatureName></SecondaryAxis></Value></Frame><Frame><Id>Frame3</Id><Value><Name>to T1</Name><Origin><Source>GeometricFeature</Source><FeatureName>planar surface 15</FeatureName></Origin><PrimaryAxis><DefinedDirection>+X</DefinedDirection><Source>GeometricFeature</Source><SourceDirection>+Z</SourceDirection><FeatureName>planar surface 15</FeatureName></PrimaryAxis><SecondaryAxis><DefinedDirection>+Y</DefinedDirection><Source>ReferenceFrame</Source><SourceDirection>+X</SourceDirection><FeatureName></FeatureName></SecondaryAxis></Value></Frame></Frames>  GraphicType=FromGeometry  MarkerShape=Sphere  MarkerSize=10  GraphicVisPropType=SimpleVisualProperties  GraphicDiffuseColor=[0.5 0.5 0.5]  GraphicSpecularColor=[0.5 0.5 0.5 1.0]  GraphicAmbientColor=[0.15 0.15 0.15 1.0]  GraphicEmissiveColor=[0.0 0.0 0.0 1.0]  GraphicShininess=75  GraphicOpacity=1.0
  Weld Joint : sm_lib/Joints/Weld Joint  JointMode=Normal  SenseConstraintForce=off  SenseConstraintForceX=off  SenseConstraintForceY=off  SenseConstraintForceZ=off  SenseConstraintTorque=off  SenseConstraintTorqueX=off  SenseConstraintTorqueY=off  SenseConstraintTorqueZ=off  SenseTotalForce=off  SenseTotalForceX=off  SenseTotalForceY=off  SenseTotalForceZ=off  SenseTotalTorque=off  SenseTotalTorqueX=off  SenseTotalTorqueY=off  SenseTotalTorqueZ=off  CompositeWrenchDir=FollowerOnBase  CompositeWrenchFrame=BaseFrame
  to T3 : PMIOPort  Side=Left
  T2 COM : PMIOPort  Port=2  Side=Left
  T2 R : PMIOPort  Port=3  Side=Right
  to T1 : PMIOPort  Port=4  Side=Right
  connections:
  to T1/RConn1 -- T2/RConn2
  T2/RConn1 -- T2 R/RConn1
  T2 COM/RConn1 -- T2/LConn1
  Weld Joint/RConn1 -- T2/LConn2
  Weld Joint/LConn1 -- to T3/RConn1

== system draft3/Thoracic Spine with rigid joints/T3 ==
  T3 : sm_lib/Body Elements/File Solid  ExtGeomFileName=C:\Users\siril\OneDrive\Desktop\TIM-Control\Matlab\Simscape models\CAD - with COM\T3_.step  UnitType=FromFile  ExtGeomFileUnits=m  StepReaderType=HEX  ExportConvexHullGeometry=off  InertiaType=CalculateFromGeometry  Mass=1  MassUnits=kg  CenterOfMass=[0 0 0]  CenterOfMassUnits=m  MomentsOfInertia=[1 1 1]  MomentsOfInertiaUnits=kg*m^2  ProductsOfInertia=[0 0 0]  ProductsOfInertiaUnits=kg*m^2  BasedOnType=Density  Density=0.99  DensityUnits=g/cm^3  DoExposeReferenceFrame=on  SerializedFrames=<Frames><Frame><Id>Frame1</Id><Value><Name>COM</Name><Origin><Source>CenterOfMassFrame</Source><FeatureName></FeatureName></Origin><PrimaryAxis><DefinedDirection>+Z</DefinedDirection><Source>ReferenceFrame</Source><SourceDirection>+Z</SourceDirection><FeatureName></FeatureName></PrimaryAxis><SecondaryAxis><DefinedDirection>+X</DefinedDirection><Source>ReferenceFrame</Source><SourceDirection>+X</SourceDirection><FeatureName></FeatureName></SecondaryAxis></Value></Frame><Frame><Id>Frame2</Id><Value><Name>to T4</Name><Origin><Source>GeometricFeature</Source><FeatureName>planar surface 5</FeatureName></Origin><PrimaryAxis><DefinedDirection>+X</DefinedDirection><Source>GeometricFeature</Source><SourceDirection>+Z</SourceDirection><FeatureName>planar surface 5</FeatureName></PrimaryAxis><SecondaryAxis><DefinedDirection>+Y</DefinedDirection><Source>ReferenceFrame</Source><SourceDirection>+X</SourceDirection><FeatureName></FeatureName></SecondaryAxis></Value></Frame><Frame><Id>Frame3</Id><Value><Name>to T2</Name><Origin><Source>GeometricFeature</Source><FeatureName>planar surface 10</FeatureName></Origin><PrimaryAxis><DefinedDirection>+X</DefinedDirection><Source>GeometricFeature</Source><SourceDirection>+Z</SourceDirection><FeatureName>planar surface 10</FeatureName></PrimaryAxis><SecondaryAxis><DefinedDirection>+Y</DefinedDirection><Source>GeometricFeature</Source><SourceDirection>+X</SourceDirection><FeatureName>segment 32</FeatureName></SecondaryAxis></Value></Frame></Frames>  GraphicType=FromGeometry  MarkerShape=Sphere  MarkerSize=10  GraphicVisPropType=SimpleVisualProperties  GraphicDiffuseColor=[0.5 0.5 0.5]  GraphicSpecularColor=[0.5 0.5 0.5 1.0]  GraphicAmbientColor=[0.15 0.15 0.15 1.0]  GraphicEmissiveColor=[0.0 0.0 0.0 1.0]  GraphicShininess=75  GraphicOpacity=1.0
  Weld Joint : sm_lib/Joints/Weld Joint  JointMode=Normal  SenseConstraintForce=off  SenseConstraintForceX=off  SenseConstraintForceY=off  SenseConstraintForceZ=off  SenseConstraintTorque=off  SenseConstraintTorqueX=off  SenseConstraintTorqueY=off  SenseConstraintTorqueZ=off  SenseTotalForce=off  SenseTotalForceX=off  SenseTotalForceY=off  SenseTotalForceZ=off  SenseTotalTorque=off  SenseTotalTorqueX=off  SenseTotalTorqueY=off  SenseTotalTorqueZ=off  CompositeWrenchDir=FollowerOnBase  CompositeWrenchFrame=BaseFrame
  to T4 : PMIOPort  Side=Left
  T3 COM : PMIOPort  Port=2  Side=Left
  T3 R : PMIOPort  Port=3  Side=Right
  to T2 : PMIOPort  Port=4  Side=Right
  connections:
  T3 COM/RConn1 -- T3/LConn1
  T3/RConn1 -- T3 R/RConn1
  to T2/RConn1 -- T3/RConn2
  to T4/RConn1 -- Weld Joint/LConn1
  Weld Joint/RConn1 -- T3/LConn2

== system draft3/Thoracic Spine with rigid joints/T4 ==
  T4 : sm_lib/Body Elements/File Solid  ExtGeomFileName=C:\Users\siril\OneDrive\Desktop\TIM-Control\Matlab\Simscape models\CAD - with COM\T4_.step  UnitType=FromFile  ExtGeomFileUnits=m  StepReaderType=HEX  ExportConvexHullGeometry=off  InertiaType=CalculateFromGeometry  Mass=1  MassUnits=kg  CenterOfMass=[0 0 0]  CenterOfMassUnits=m  MomentsOfInertia=[1 1 1]  MomentsOfInertiaUnits=kg*m^2  ProductsOfInertia=[0 0 0]  ProductsOfInertiaUnits=kg*m^2  BasedOnType=Density  Density=0.99  DensityUnits=g/cm^3  DoExposeReferenceFrame=on  SerializedFrames=<Frames><Frame><Id>Frame1</Id><Value><Name>COM</Name><Origin><Source>CenterOfMassFrame</Source><FeatureName></FeatureName></Origin><PrimaryAxis><DefinedDirection>+Z</DefinedDirection><Source>ReferenceFrame</Source><SourceDirection>+Z</SourceDirection><FeatureName></FeatureName></PrimaryAxis><SecondaryAxis><DefinedDirection>+X</DefinedDirection><Source>ReferenceFrame</Source><SourceDirection>+X</SourceDirection><FeatureName></FeatureName></SecondaryAxis></Value></Frame><Frame><Id>Frame2</Id><Value><Name>to T5</Name><Origin><Source>GeometricFeature</Source><FeatureName>planar surface 5</FeatureName></Origin><PrimaryAxis><DefinedDirection>+X</DefinedDirection><Source>GeometricFeature</Source><SourceDirection>+Z</SourceDirection><FeatureName>planar surface 5</FeatureName></PrimaryAxis><SecondaryAxis><DefinedDirection>+Y</DefinedDirection><Source>GeometricFeature</Source><SourceDirection>+X</SourceDirection><FeatureName>segment 8</FeatureName></SecondaryAxis></Value></Frame><Frame><Id>Frame3</Id><Value><Name>to T3</Name><Origin><Source>GeometricFeature</Source><FeatureName>planar surface 17</FeatureName></Origin><PrimaryAxis><DefinedDirection>+X</DefinedDirection><Source>GeometricFeature</Source><SourceDirection>+Z</SourceDirection><FeatureName>planar surface 17</FeatureName></PrimaryAxis><SecondaryAxis><DefinedDirection>+Y</DefinedDirection><Source>GeometricFeature</Source><SourceDirection>+X</SourceDirection><FeatureName>segment 46</FeatureName></SecondaryAxis></Value></Frame></Frames>  GraphicType=FromGeometry  MarkerShape=Sphere  MarkerSize=10  GraphicVisPropType=SimpleVisualProperties  GraphicDiffuseColor=[0.5 0.5 0.5]  GraphicSpecularColor=[0.5 0.5 0.5 1.0]  GraphicAmbientColor=[0.15 0.15 0.15 1.0]  GraphicEmissiveColor=[0.0 0.0 0.0 1.0]  GraphicShininess=75  GraphicOpacity=1.0
  Weld Joint : sm_lib/Joints/Weld Joint  JointMode=Normal  SenseConstraintForce=off  SenseConstraintForceX=off  SenseConstraintForceY=off  SenseConstraintForceZ=off  SenseConstraintTorque=off  SenseConstraintTorqueX=off  SenseConstraintTorqueY=off  SenseConstraintTorqueZ=off  SenseTotalForce=off  SenseTotalForceX=off  SenseTotalForceY=off  SenseTotalForceZ=off  SenseTotalTorque=off  SenseTotalTorqueX=off  SenseTotalTorqueY=off  SenseTotalTorqueZ=off  CompositeWrenchDir=FollowerOnBase  CompositeWrenchFrame=BaseFrame
  to T5 : PMIOPort  Side=Left
  T4 COM : PMIOPort  Port=2  Side=Left
  T4 R : PMIOPort  Port=3  Side=Right
  to T3 : PMIOPort  Port=4  Side=Right
  connections:
  to T3/RConn1 -- T4/RConn2
  T4/RConn1 -- T4 R/RConn1
  T4 COM/RConn1 -- T4/LConn1
  to T5/RConn1 -- Weld Joint/LConn1
  Weld Joint/RConn1 -- T4/LConn2

== system draft3/Thoracic Spine with rigid joints/T5 ==
  T5 : sm_lib/Body Elements/File Solid  ExtGeomFileName=C:\Users\siril\OneDrive\Desktop\TIM-Control\Matlab\Simscape models\CAD - with COM\T5_.step  UnitType=FromFile  ExtGeomFileUnits=m  StepReaderType=HEX  ExportConvexHullGeometry=off  InertiaType=CalculateFromGeometry  Mass=1  MassUnits=kg  CenterOfMass=[0 0 0]  CenterOfMassUnits=m  MomentsOfInertia=[1 1 1]  MomentsOfInertiaUnits=kg*m^2  ProductsOfInertia=[0 0 0]  ProductsOfInertiaUnits=kg*m^2  BasedOnType=Density  Density=0.99  DensityUnits=g/cm^3  DoExposeReferenceFrame=on  SerializedFrames=<Frames><Frame><Id>Frame1</Id><Value><Name>F1</Name><Origin><Source>CenterOfMassFrame</Source><FeatureName></FeatureName></Origin><PrimaryAxis><DefinedDirection>+Z</DefinedDirection><Source>ReferenceFrame</Source><SourceDirection>+Z</SourceDirection><FeatureName></FeatureName></PrimaryAxis><SecondaryAxis><DefinedDirection>+X</DefinedDirection><Source>ReferenceFrame</Source><SourceDirection>+X</SourceDirection><FeatureName></FeatureName></SecondaryAxis></Value></Frame><Frame><Id>Frame2</Id><Value><Name>to T6</Name><Origin><Source>GeometricFeature</Source><FeatureName>planar surface 6</FeatureName></Origin><PrimaryAxis><DefinedDirection>+Y</DefinedDirection><Source>GeometricFeature</Source><SourceDirection>+Z</SourceDirection><FeatureName>segment 19</FeatureName></PrimaryAxis><SecondaryAxis><DefinedDirection>+Z</DefinedDirection><Source>GeometricFeature</Source><SourceDirection>+X</SourceDirection><FeatureName>segment 17</FeatureName></SecondaryAxis></Value></Frame><Frame><Id>Frame3</Id><Value><Name>to T4</Name><Origin><Source>GeometricFeature</Source><FeatureName>planar surface 13</FeatureName></Origin><PrimaryAxis><DefinedDirection>+X</DefinedDirection><Source>GeometricFeature</Source><SourceDirection>+Z</SourceDirection><FeatureName>planar surface 13</FeatureName></PrimaryAxis><SecondaryAxis><DefinedDirection>+Y</DefinedDirection><Source>GeometricFeature</Source><SourceDirection>+X</SourceDirection><FeatureName>segment 34</FeatureName></SecondaryAxis></Value></Frame></Frames>  GraphicType=FromGeometry  MarkerShape=Sphere  MarkerSize=10  GraphicVisPropType=SimpleVisualProperties  GraphicDiffuseColor=[0.5 0.5 0.5]  GraphicSpecularColor=[0.5 0.5 0.5 1.0]  GraphicAmbientColor=[0.15 0.15 0.15 1.0]  GraphicEmissiveColor=[0.0 0.0 0.0 1.0]  GraphicShininess=75  GraphicOpacity=1.0
  Weld Joint : sm_lib/Joints/Weld Joint  JointMode=Normal  SenseConstraintForce=off  SenseConstraintForceX=off  SenseConstraintForceY=off  SenseConstraintForceZ=off  SenseConstraintTorque=off  SenseConstraintTorqueX=off  SenseConstraintTorqueY=off  SenseConstraintTorqueZ=off  SenseTotalForce=off  SenseTotalForceX=off  SenseTotalForceY=off  SenseTotalForceZ=off  SenseTotalTorque=off  SenseTotalTorqueX=off  SenseTotalTorqueY=off  SenseTotalTorqueZ=off  CompositeWrenchDir=FollowerOnBase  CompositeWrenchFrame=BaseFrame
  to T6 : PMIOPort  Side=Left
  T5 COM : PMIOPort  Port=2  Side=Left
  T5 R : PMIOPort  Port=3  Side=Right
  to T4 : PMIOPort  Port=4  Side=Right
  connections:
  T5 COM/RConn1 -- T5/LConn1
  T5/RConn1 -- T5 R/RConn1
  to T4/RConn1 -- T5/RConn2
  to T6/RConn1 -- Weld Joint/LConn1
  Weld Joint/RConn1 -- T5/LConn2

== system draft3/Thoracic Spine with rigid joints/T6 ==
  T6 : sm_lib/Body Elements/File Solid  ExtGeomFileName=C:\Users\siril\OneDrive\Desktop\TIM-Control\Matlab\Simscape models\CAD - with COM\T6_.step  UnitType=FromFile  ExtGeomFileUnits=m  StepReaderType=HEX  ExportConvexHullGeometry=off  InertiaType=CalculateFromGeometry  Mass=1  MassUnits=kg  CenterOfMass=[0 0 0]  CenterOfMassUnits=m  MomentsOfInertia=[1 1 1]  MomentsOfInertiaUnits=kg*m^2  ProductsOfInertia=[0 0 0]  ProductsOfInertiaUnits=kg*m^2  BasedOnType=Density  Density=0.99  DensityUnits=g/cm^3  DoExposeReferenceFrame=on  SerializedFrames=<Frames><Frame><Id>Frame1</Id><Value><Name>COM</Name><Origin><Source>CenterOfMassFrame</Source><FeatureName></FeatureName></Origin><PrimaryAxis><DefinedDirection>+Z</DefinedDirection><Source>ReferenceFrame</Source><SourceDirection>+Z</SourceDirection><FeatureName></FeatureName></PrimaryAxis><SecondaryAxis><DefinedDirection>+X</DefinedDirection><Source>ReferenceFrame</Source><SourceDirection>+X</SourceDirection><FeatureName></FeatureName></SecondaryAxis></Value></Frame><Frame><Id>Frame2</Id><Value><Name>to T7</Name><Origin><Source>GeometricFeature</Source><FeatureName>planar surface 5</FeatureName></Origin><PrimaryAxis><DefinedDirection>+Y</DefinedDirection><Source>GeometricFeature</Source><SourceDirection>+Z</SourceDirection><FeatureName>segment 12</FeatureName></PrimaryAxis><SecondaryAxis><DefinedDirection>+Z</DefinedDirection><Source>GeometricFeature</Source><SourceDirection>+X</SourceDirection><FeatureName>segment 9</FeatureName></SecondaryAxis></Value></Frame><Frame><Id>Frame3</Id><Value><Name>to T5</Name><Origin><Source>GeometricFeature</Source><FeatureName>segment 27</FeatureName></Origin><PrimaryAxis><DefinedDirection>-X</DefinedDirection><Source>GeometricFeature</Source><SourceDirection>+Z</SourceDirection><FeatureName>planar surface 10</FeatureName></PrimaryAxis><SecondaryAxis><DefinedDirection>+Y</DefinedDirection><Source>ReferenceFrame</Source><SourceDirection>+X</SourceDirection><FeatureName></FeatureName></SecondaryAxis></Value></Frame></Frames>  GraphicType=FromGeometry  MarkerShape=Sphere  MarkerSize=10  GraphicVisPropType=SimpleVisualProperties  GraphicDiffuseColor=[0.5 0.5 0.5]  GraphicSpecularColor=[0.5 0.5 0.5 1.0]  GraphicAmbientColor=[0.15 0.15 0.15 1.0]  GraphicEmissiveColor=[0.0 0.0 0.0 1.0]  GraphicShininess=75  GraphicOpacity=1.0
  Weld Joint : sm_lib/Joints/Weld Joint  JointMode=Normal  SenseConstraintForce=off  SenseConstraintForceX=off  SenseConstraintForceY=off  SenseConstraintForceZ=off  SenseConstraintTorque=off  SenseConstraintTorqueX=off  SenseConstraintTorqueY=off  SenseConstraintTorqueZ=off  SenseTotalForce=off  SenseTotalForceX=off  SenseTotalForceY=off  SenseTotalForceZ=off  SenseTotalTorque=off  SenseTotalTorqueX=off  SenseTotalTorqueY=off  SenseTotalTorqueZ=off  CompositeWrenchDir=FollowerOnBase  CompositeWrenchFrame=BaseFrame
  to T7 : PMIOPort  Side=Left
  T6 COM : PMIOPort  Port=2  Side=Left
  T6 R : PMIOPort  Port=3  Side=Right
  to T5 : PMIOPort  Port=4  Side=Right
  connections:
  to T5/RConn1 -- T6/RConn2
  T6/RConn1 -- T6 R/RConn1
  T6 COM/RConn1 -- T6/LConn1
  to T7/RConn1 -- Weld Joint/LConn1
  Weld Joint/RConn1 -- T6/LConn2
